simulink model "PV"  (R2026a)
settings: Solver=VariableStepAuto
libraries: fl_lib x2, nesl_utility x2

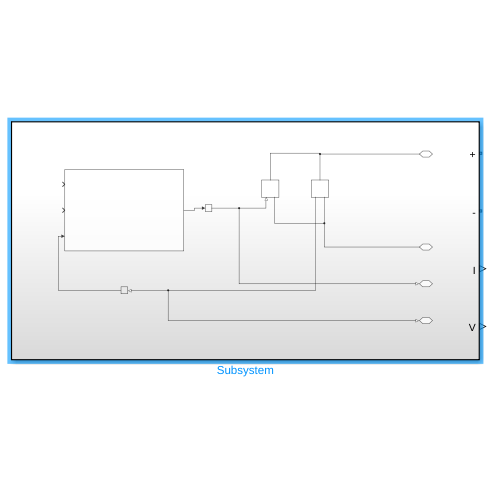
[thumbnail: Simulink's stored preview of the top-level diagram]
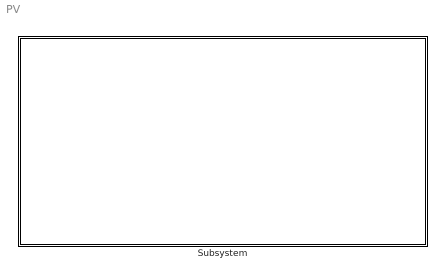
== system PV ==
  Subsystem : Subsystem

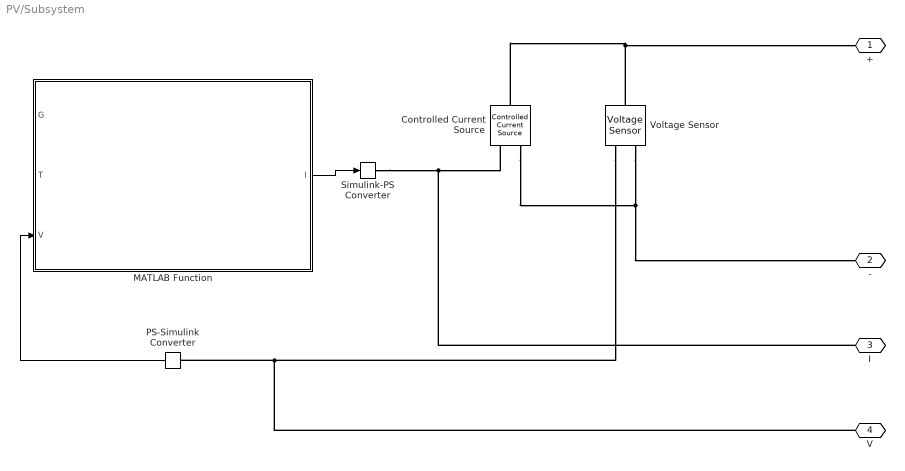
== system PV/Subsystem ==
  Controlled Current Source : fl_lib/Electrical/Electrical Sources/Controlled Current Source
  MATLAB Function : MATLAB Function  TreatAsAtomicUnit=on
  PS-Simulink Converter : nesl_utility/PS-Simulink Converter  PhysicalDomain=network_engine_domain  SubClassName=ps_output  LeftPortType=input  RightPortType=output  PseudoPeriodic=off  Frequencies=[]  VectorFormat=inherit  Unit=inherit  AffineConversion=off
  Simulink-PS Converter : nesl_utility/Simulink-PS Converter  PhysicalDomain=network_engine_domain  SubClassName=ps_input  LeftPortType=input  RightPortType=output  PseudoPeriodic=off  Frequencies=[]  NoiseDistribution=none  NoiseParameters=[]  Unit=1  AffineConversion=off  FilteringAndDerivatives=provide  SimscapeFilterOrder=1  InputFilterTimeConstant=0.001  UdotUserProvided=0
  Voltage Sensor : fl_lib/Electrical/Electrical Sensors/Voltage Sensor
  + : PMIOPort  Side=Right
  - : PMIOPort  Port=2  Side=Right
  I : PMIOPort  Port=3  Side=Right
  V : PMIOPort  Port=4  Side=Right
  wires:
  MATLAB Function/1(I) -> Simulink-PS Converter/1
  PS-Simulink Converter/1 -> MATLAB Function/3(V)
  connections:
  Simulink-PS Converter/RConn1 -- I/RConn1 -- Controlled Current Source/RConn1
  Voltage Sensor/RConn1 -- V/RConn1 -- PS-Simulink Converter/LConn1
  Controlled Current Source/RConn2 -- -/RConn1 -- Voltage Sensor/RConn2
  Controlled Current Source/LConn1 -- Voltage Sensor/LConn1 -- +/RConn1

== matlab function PV/Subsystem/MATLAB Function ==
  data: G input; I output; T input; V input
function I = modelo_pv(G, T, V)

    % ---- Parâmetros do datasheet (painel monocristalino, ~50W) ----
    Isc_ref = 3.14;    % A
    Voc_ref = 21.4;    % V
    Kv = -0.080;       % V/°C
    Ki = 0.0024;       % A/°C
    Ns = 36;           % número de células em série

    k = 1.3806e-23; % Constante de Boltzmann
    q = 1.6022e-19; % Carga do elétron
    a = 1.2;        % Fator de idealidade do diodo

    T_kelvin = T + 273.15;
    T_ref = 25 + 273.15;
    G_ref = 1000;

    % proteção: limita V a uma faixa fisicamente plausível
    V = max(min(V, 1.5*Voc_ref), -1);

    % 1. Corrente Fotogerada (Iph)
    Iph = (Isc_ref + Ki * (T_kelvin - T_ref)) * (G / G_ref);

    % 2. Corrente de Saturação do Diodo (Irs e I0)
    Irs = Isc_ref / (exp((q * Voc_ref) / (Ns * k * a * T_ref)) - 1);
    I0 = Irs * (T_kelvin / T_ref)^3 * exp((q * 1.12 / (a * k)) * (1/T_ref - 1/T_kelvin));

    % 3. Corrente de Saída
    expoente = min((q * V) / (Ns * k * a * T_kelvin), 80);
    Id = I0 * (exp(expoente) - 1);

    I = Iph - Id;

    if I < 0
        I = 0;
    end
end
